simulink model "CarModel_MPCCtrl"  (R2022b)
settings: Solver=VariableStepAuto  StartTime=0.0  StopTime=Tf  RelTol=1e-3
values from neighbouring files (symbols this model uses):
  a = -DenM(2)    [Setup_Ctrl.m]
  du_max = 1    [Setup_Ctrl.m]
  g = NumM(1)    [Setup_Ctrl.m]
  H_p = 10    [Setup_Ctrl.m]
  Ts = 4    [Setup_Ctrl.m]    (also in Setup_Id.m = 0.5)
  u_max = 1    [Setup_Ctrl.m]
undefined symbols (not defined in the file or in its folder): magnitude
libraries: simulink x4
settings Model: Creator=rvilanova  LastModifiedBy=rvilanova

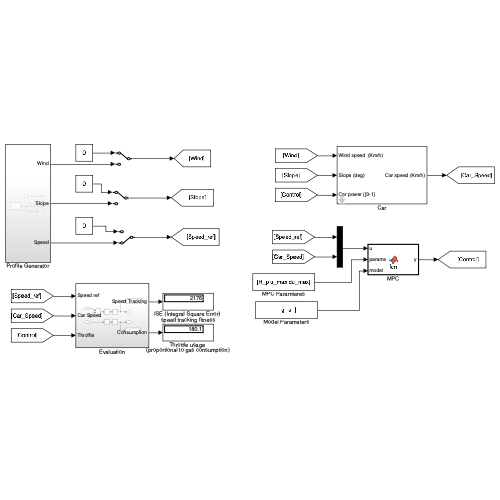
[thumbnail: Simulink's stored preview of the top-level diagram]
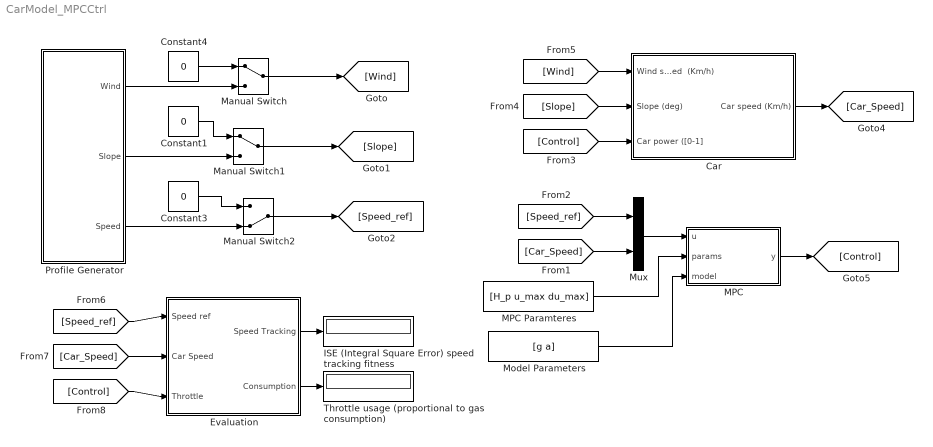
== system CarModel_MPCCtrl ==
  Car : Subsystem  mask{M=1000}
      mask prompts: M "Pes del vehicle"
  Constant1 : Constant  Value=0
  Constant3 : Constant  Value=0
  Constant4 : Constant  Value=0
  Evaluation : Subsystem
  ISE (Integral Square Error) speed tracking fitness : Display
  MPC : MATLAB Function  TreatAsAtomicUnit=on
  MPC Paramteres : Constant  Value=[H_p u_max du_max]
  Manual Switch : ManualSwitch
  Manual Switch1 : ManualSwitch
  Manual Switch2 : ManualSwitch  CurrentSetting=0
  Model Parameters : Constant  Value=[g a]
  Mux : Mux  Inputs=2
  Profile Generator : Subsystem
  Throttle usage (proportional to gas consumption) : Display
  wires:
  Manual Switch1/1 -> [Slope]
  Profile Generator/3(Speed) -> Manual Switch2/2
  Profile Generator/1(Wind) -> Manual Switch/2
  Manual Switch/1 -> [Wind]
  Constant4/1 -> Manual Switch/1
  Profile Generator/2(Slope) -> Manual Switch1/2
  Constant3/1 -> Manual Switch2/1
  Constant1/1 -> Manual Switch1/1
  [Slope] -> Car/2(Slope (deg))
  Car/1(Car speed (Km/h)) -> [Car_Speed]
  [Wind] -> Car/1(Wind speed  (Km/h))
  [Speed_ref] -> Mux/1
  Mux/1 -> MPC/1(u)
  MPC Paramteres/1 -> MPC/2(params)
  MPC/1(y) -> [Control]
  [Car_Speed] -> Mux/2
  Model Parameters/1 -> MPC/3(model)
  [Control] -> Car/3(Car power ([0-1])
  Manual Switch2/1 -> [Speed_ref]
  [Speed_ref] -> Evaluation/1(Speed ref)
  [Car_Speed] -> Evaluation/2(Car Speed)
  [Control] -> Evaluation/3(Throttle)
  Evaluation/1(Speed Tracking) -> ISE (Integral Square Error) speed tracking fitness/1
  Evaluation/2(Consumption) -> Throttle usage (proportional to gas consumption)/1

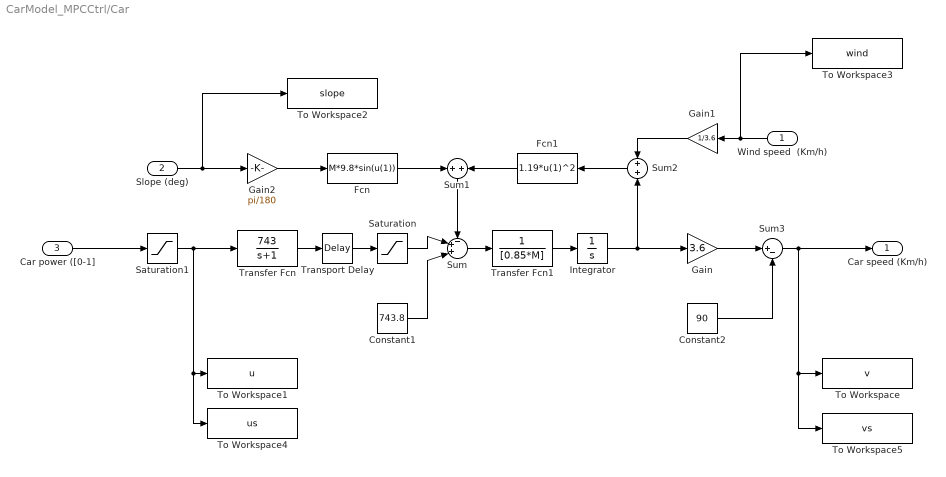
== system CarModel_MPCCtrl/Car ==
  Wind speed  (Km/h) : Inport
  Slope (deg) : Inport  Port=2
  Car power ([0-1] : Inport  Port=3
  Constant1 : Constant  Value=743.8
  Constant2 : Constant  Value=90
  Fcn : Fcn  Expr=M*9.8*sin(u(1))
  Fcn1 : Fcn  Expr=1.19*u(1)^2
  Gain : Gain  Gain=3.6
  Gain1 : Gain  Gain=1/3.6
  Gain2 : Gain  Gain=pi/180
  Integrator : Integrator  InitialCondition=25
  Saturation : Saturate  UpperLimit=3000  LowerLimit=-3000
  Saturation1 : Saturate  UpperLimit=1  LowerLimit=-1
  Sum : Sum  Inputs=-++|  InputSameDT=on  SaturateOnIntegerOverflow=on  OutDataTypeStr=Inherit: Same as first input
  Sum1 : Sum  InputSameDT=on  SaturateOnIntegerOverflow=on  OutDataTypeStr=Inherit: Same as first input
  Sum2 : Sum  Inputs=+|+  InputSameDT=on  SaturateOnIntegerOverflow=on  OutDataTypeStr=Inherit: Same as first input
  Sum3 : Sum  Inputs=|+-  InputSameDT=on  SaturateOnIntegerOverflow=on  OutDataTypeStr=Inherit: Same as first input
  To Workspace : ToWorkspace  VariableName=v  SaveFormat=Timeseries  SampleTime=-1
  To Workspace1 : ToWorkspace  VariableName=u  SaveFormat=Timeseries  SampleTime=-1
  To Workspace2 : ToWorkspace  VariableName=slope  SaveFormat=Timeseries  SampleTime=-1
  To Workspace3 : ToWorkspace  VariableName=wind  SaveFormat=Timeseries  SampleTime=-1
  To Workspace4 : ToWorkspace  VariableName=us  SaveFormat=Timeseries  SampleTime=Ts
  To Workspace5 : ToWorkspace  VariableName=vs  SaveFormat=Timeseries  SampleTime=Ts
  Transfer Fcn : TransferFcn  Numerator=[743]  Denominator=[1 1]
  Transfer Fcn1 : TransferFcn  Denominator=[0.85*M]
  Transport Delay : TransportDelay  DelayTime=0.3
  Car speed (Km/h) : Outport
  wires:
  Slope (deg)/1 -> To Workspace2/1, Gain2/1
  Gain2/1 -> Fcn/1
  Gain1/1 -> Sum2/1
  Wind speed  (Km/h)/1 -> To Workspace3/1, Gain1/1
  Transfer Fcn/1 -> Transport Delay/1
  Transport Delay/1 -> Saturation/1
  Sum/1 -> Transfer Fcn1/1
  Transfer Fcn1/1 -> Integrator/1
  Fcn1/1 -> Sum1/2
  Sum2/1 -> Fcn1/1
  Sum1/1 -> Sum/1
  Fcn/1 -> Sum1/1
  Integrator/1 -> Gain/1, Sum2/2
  Car power ([0-1]/1 -> Saturation1/1
  Saturation/1 -> Sum/2
  Constant1/1 -> Sum/3
  Gain/1 -> Sum3/1
  Sum3/1 -> To Workspace5/1, To Workspace/1, Car speed (Km/h)/1
  Constant2/1 -> Sum3/2
  Saturation1/1 -> To Workspace4/1, To Workspace1/1, Transfer Fcn/1

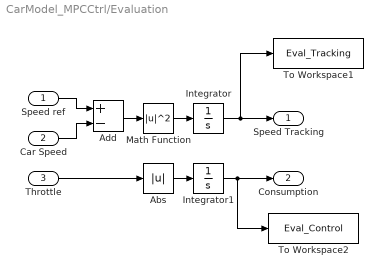
== system CarModel_MPCCtrl/Evaluation ==
  Speed ref : Inport
  Car Speed : Inport  Port=2
  Throttle : Inport  Port=3
  Abs : Abs  SaturateOnIntegerOverflow=off
  Add : Sum  Inputs=+-
  Integrator : Integrator
  Integrator1 : Integrator
  Math Function : Math  Operator=magnitude^2
  To Workspace1 : ToWorkspace  VariableName=Eval_Tracking  SaveFormat=Timeseries  SampleTime=-1
  To Workspace2 : ToWorkspace  VariableName=Eval_Control  SaveFormat=Timeseries  SampleTime=-1
  Speed Tracking : Outport
  Consumption : Outport  Port=2
  wires:
  Throttle/1 -> Abs/1
  Integrator1/1 -> To Workspace2/1, Consumption/1
  Integrator/1 -> To Workspace1/1, Speed Tracking/1
  Car Speed/1 -> Add/2
  Add/1 -> Math Function/1
  Speed ref/1 -> Add/1
  Math Function/1 -> Integrator/1
  Abs/1 -> Integrator1/1

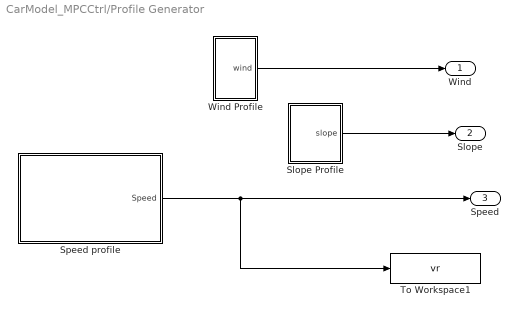
== system CarModel_MPCCtrl/Profile Generator ==
  Slope Profile : Subsystem
  Speed profile : Subsystem
  To Workspace1 : ToWorkspace  VariableName=vr  SaveFormat=Timeseries  SampleTime=-1
  Wind Profile : Subsystem
  Wind : Outport
  Slope : Outport  Port=2
  Speed : Outport  Port=3
  wires:
  Slope Profile/1(slope) -> Slope/1
  Wind Profile/1(wind) -> Wind/1
  Speed profile/1(Speed) -> Speed/1, To Workspace1/1

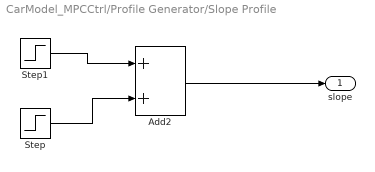
== system CarModel_MPCCtrl/Profile Generator/Slope Profile ==
  Add2 : Sum
  Step : Step  Time=400  After=5*(pi/180)  SampleTime=0
  Step1 : Step  Time=350  After=-5*(pi/180)  SampleTime=0
  slope : Outport
  wires:
  Step1/1 -> Add2/1
  Step/1 -> Add2/2
  Add2/1 -> slope/1

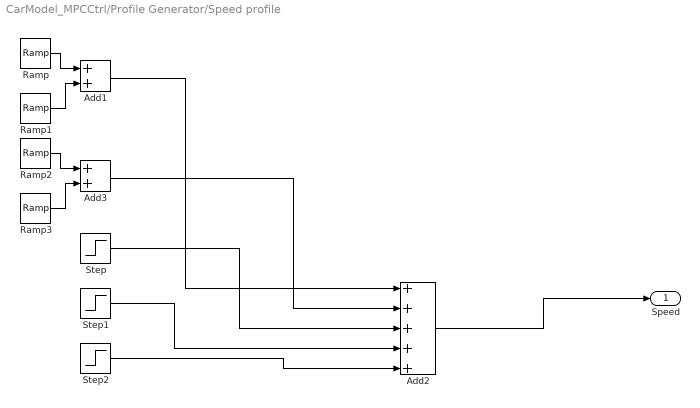
== system CarModel_MPCCtrl/Profile Generator/Speed profile ==
  Add1 : Sum
  Add2 : Sum  Inputs=+++++
  Add3 : Sum
  Ramp : simulink/Sources/Ramp  slope=0.5  start=20  InitialOutput=0
  Ramp1 : simulink/Sources/Ramp  slope=-0.5  start=60  InitialOutput=0
  Ramp2 : simulink/Sources/Ramp  slope=-0.5  start=260  InitialOutput=0
  Ramp3 : simulink/Sources/Ramp  slope=0.5  start=300  InitialOutput=0
  Step : Step  Time=500  After=-10  SampleTime=0
  Step1 : Step  Time=600  After=20  SampleTime=0
  Step2 : Step  Time=700  After=-10  SampleTime=0
  Speed : Outport
  wires:
  Ramp3/1 -> Add3/2
  Add3/1 -> Add2/2
  Step2/1 -> Add2/5
  Step1/1 -> Add2/4
  Add2/1 -> Speed/1
  Ramp2/1 -> Add3/1
  Ramp/1 -> Add1/1
  Ramp1/1 -> Add1/2
  Add1/1 -> Add2/1
  Step/1 -> Add2/3

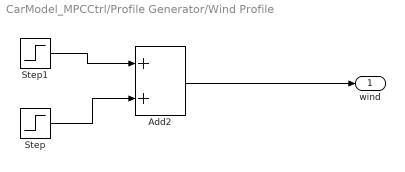
== system CarModel_MPCCtrl/Profile Generator/Wind Profile ==
  Add2 : Sum
  Step : Step  Time=150  After=-20  SampleTime=0
  Step1 : Step  Time=100  After=20  SampleTime=0
  wind : Outport
  wires:
  Step1/1 -> Add2/1
  Step/1 -> Add2/2
  Add2/1 -> wind/1

== matlab function CarModel_MPCCtrl/MPC ==
  data: u input; y output; params input; model input
function y = fcn(u, params, model)

% Extract paramters from input #1
y_sp=u(1);
y_0=u(2);

% Extract paramters from input #2
H_p = params(1);   
u_max=params(2);
du_max=params(3);

% Extract paramters from input #3
% Prediction model
g=model(1);
a=model(2);

% Prediction elements for QP problem
L=zeros(H_p,H_p);
for j=1:H_p
    for k=1:j 
        L(j,k)=g*a^(j-k);
    end
end


% Elements of the Qp problem
H=zeros(H_p,H_p);
for k=1:H_p
    H=H+L(k,:)'*L(k,:);
end

f=zeros(1,H_p);
for k=1:H_p
    f=f+(a^k*y_0-y_sp)*L(k,:);
end

% Amplitude saturation constraints

A1=[eye(H_p,H_p); -eye(H_p,H_p)];
b1=u_max*ones(2*H_p,1);


% Increment saturation constraints
D=zeros(H_p-1,H_p);
for k=1:H_p-1
    D(k,k:k+1)=[1 -1];
end
A2=[D; -D];
b2=du_max*ones(2*(H_p-1),1);

% Inequality constraints of the QP problem 
A=[A1 ; A2];
b=[b1 ; b2];


% Final termination constarint
Aeq=L(H_p,:);
beq=y_sp-a^H_p*y_0;

%% SOLUTION 

% Unconstrained problem
%u_o=quadprog(H,f);

% Constrained problem
%

LB=[];
UB=[];
x0=zeros(1,H_p);

options = optimoptions('quadprog','Algorithm','active-set');
% u_o=quadprog(H,f,A,b,Aeq,beq,LB,UB,x0,options);
u_o=quadprog(H,f,[],[],[],[],[],[],x0,options);



% Receding Horizon, just need the first element
y = u_o(1);
